simulink model "ParallelAndSeriesModulesSimulation"  (R2016a)
settings: Solver=VariableStepAuto  StartTime=0.0  StopTime=0.25  RelTol=1e-3
libraries: powerlib x17, powerlib_meascontrol x10, electricdrivelib x2
settings Model: Creator=kkfrk  LastModifiedBy=mesutto

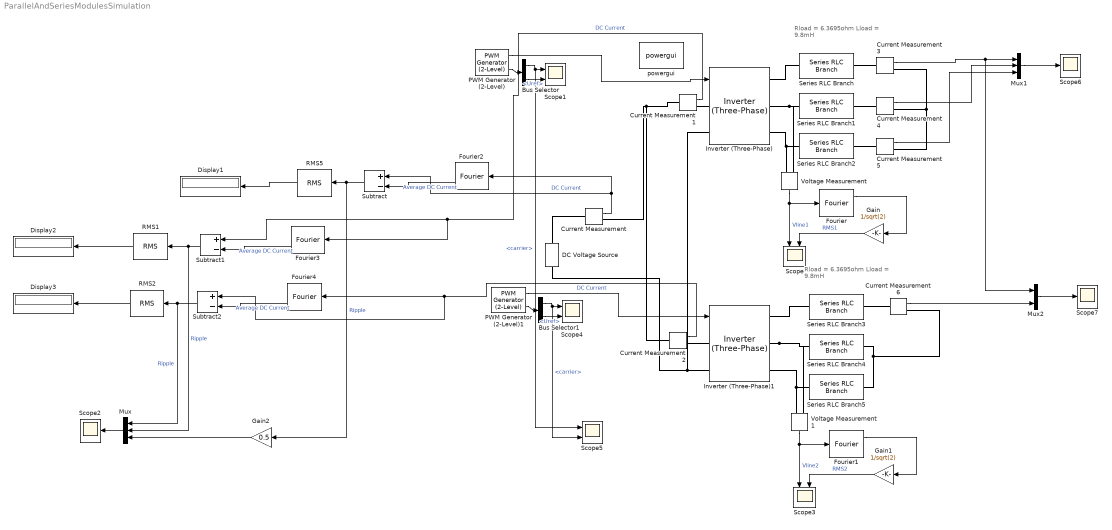
== system ParallelAndSeriesModulesSimulation ==
  note: Rload = 6.3695ohm
      | Lload = 9.8mH
  note: Rload = 6.3695ohm
      | Lload = 9.8mH
  Bus Selector : BusSelector  OutputSignals=carrier,Uref
  Bus Selector1 : BusSelector  OutputSignals=carrier,Uref
  Current Measurement{,1..6} (7 alike) : powerlib/Measurements/Current Measurement  PhasorSimulation=off  OutputType=Complex  PSBequivalent=0
  DC Voltage Source : powerlib/Electrical Sources/DC Voltage Source  Amplitude=400  Measurements=None
  Display1 : Display
  Display2 : Display
  Display3 : Display
  Fourier : powerlib_meascontrol/Measurements/Fourier  Freq=50  n=1  InInit=[0, 0]  Ts=0
  Fourier1 : powerlib_meascontrol/Measurements/Fourier  Freq=50  n=1  InInit=[0, 0]  Ts=0
  Fourier2 : powerlib_meascontrol/Measurements/Fourier  Freq=50  n=0  InInit=[0, 0]  Ts=0
  Fourier3 : powerlib_meascontrol/Measurements/Fourier  Freq=50  n=0  InInit=[0, 0]  Ts=0
  Fourier4 : powerlib_meascontrol/Measurements/Fourier  Freq=50  n=0  InInit=[0, 0]  Ts=0
  Gain : Gain  Gain=1/sqrt(2)
  Gain1 : Gain  Gain=1/sqrt(2)
  Gain2 : Gain  Gain=0.5
  Inverter (Three-Phase) : electricdrivelib/Fundamental Drive Blocks/Inverter (Three-Phase)  OverrideUsingVariant=Detailed  detailLevel=Detailed  driveType=Field-oriented control  Ts=2e-6  SnubberResistance=10e3  SnubberCapacitance=inf  Device=IGBT / Diodes  Ron=1e-3  ForwardVoltages=[1.2,1.2]  GTOparameters=[1e-6,2e-6]  IGBTparameters=[1e-6,2e-6]  Measurements=All voltages and currents  converterType=Inverter  SourceFrequency=60  ReferenceFrame=Rotor  dqInductances=[8.5e-3,8.5e-3]  Inductance=8.5e-3  Ls=0  Resistance=0.2  Flux=0.175  Stator_sm=[2.01e-3,4.289e-4,4.477e-3,1.354e-3]  Stator_im=[14.85e-3,0.3027e-3]  Rotor=[9.295e-3,0.3027e-3]  Lm=10.46e-3  p=4
      settings: AttributesFormatString=%<BlockChoice>
  Inverter (Three-Phase)1 : electricdrivelib/Fundamental Drive Blocks/Inverter (Three-Phase)  OverrideUsingVariant=Detailed  detailLevel=Detailed  driveType=Field-oriented control  Ts=2e-6  SnubberResistance=10e3  SnubberCapacitance=inf  Device=IGBT / Diodes  Ron=1e-3  ForwardVoltages=[1.2,1.2]  GTOparameters=[1e-6,2e-6]  IGBTparameters=[1e-6,2e-6]  Measurements=All voltages and currents  converterType=Inverter  SourceFrequency=60  ReferenceFrame=Rotor  dqInductances=[8.5e-3,8.5e-3]  Inductance=8.5e-3  Ls=0  Resistance=0.2  Flux=0.175  Stator_sm=[2.01e-3,4.289e-4,4.477e-3,1.354e-3]  Stator_im=[14.85e-3,0.3027e-3]  Rotor=[9.295e-3,0.3027e-3]  Lm=10.46e-3  p=4
      settings: AttributesFormatString=%<BlockChoice>
  Mux : Mux  Inputs=3
  Mux1 : Mux  Inputs=3
  Mux2 : Mux  Inputs=2
  PWM Generator (2-Level) : powerlib_meascontrol/Pulse & Signal Generators/PWM Generator (2-Level)  ModulatorType=Three-phase bridge (6 pulses)  ModulatorMode=Unsynchronized  Fc=1000  Pc=0  nF=27  MinMax="[ -1  1 ]"  SamplingTechnique=Natural  ModulatingSignals=on  m=0.8  Freq=50  Phase=0  Ts=0  ShowCarrierOutport=on
  PWM Generator (2-Level)1 : powerlib_meascontrol/Pulse & Signal Generators/PWM Generator (2-Level)  ModulatorType=Three-phase bridge (6 pulses)  ModulatorMode=Unsynchronized  Fc=1000  Pc=90  nF=27  MinMax="[ -1  1 ]"  SamplingTechnique=Natural  ModulatingSignals=on  m=0.8  Freq=50  Phase=0  Ts=0  ShowCarrierOutport=on
  RMS1 : powerlib_meascontrol/Measurements/RMS  TrueRMS=on  Freq=50  RMSInit=25  Ts=10e-6
  RMS2 : powerlib_meascontrol/Measurements/RMS  TrueRMS=on  Freq=50  RMSInit=25  Ts=10e-6
  RMS5 : powerlib_meascontrol/Measurements/RMS  TrueRMS=on  Freq=50  RMSInit=25  Ts=10e-6
  Scope{,1,3..5} (5 alike) : Scope  NumInputPorts=2
  Scope2 : Scope
  Scope6 : Scope
  Scope7 : Scope
  Series RLC Branch{,1..5} (6 alike) : powerlib/Elements/Series RLC Branch  LConnTagsString=__new0  RConnTagsString=__new0  BranchType=RLC  Resistance=6.3695  Inductance=9.8e-3  SetiL0=off  InitialCurrent=0  Capacitance=0  Setx0=off  InitialVoltage=0  Measurements=None
  Subtract : Sum  Inputs=+-
  Subtract1 : Sum  Inputs=+-
  Subtract2 : Sum  Inputs=+-
  Voltage Measurement : powerlib/Measurements/Voltage Measurement  PhasorSimulation=off  OutputType=Complex  PSBequivalent=0
  Voltage Measurement1 : powerlib/Measurements/Voltage Measurement  PhasorSimulation=off  OutputType=Complex  PSBequivalent=0
  powergui : powerlib/powergui  Priority=1  SimulationMode=Discrete  SolverType=Tustin/Backward Euler (TBE)  SampleTime=10e-6  frequency=60  SPID=off  DisableSnubberDevices=off  DisableRonSwitches=off  DisableVfSwitches=off  SwTol=0  DisplayEquations=off  Interpol=off  ExternalGateDelay=off  methode=off  Ts=10  FunctionMessages=off  echomessages=off  HookPort=off  EnableUseOfTLC=off  x0status=blocks  frequencyindice=0  Pbase=100e6  ErrMax=1e-4  Iterations=50  UnitsV=kV  UnitsW=MW  buscounter=0  RestoreLinks=warning  ResistiveCurrentMeasurement=off  Frange=[0:2:500]  Ylog=off  Xlog=on  ShowGrid=off  save=off  variable=ZData  structure=0  ZoomFFT=off  StartTime=0.0  cycles=1  DisplayStyle=1  fundamental=60  FreqAxis=off  MaxFrequency=1000  frequencyindicesteady=1  RmsSteady=1  display=off
  wires:
  Voltage Measurement/1 -> Scope/1, Fourier/1  "Vline1"
  PWM Generator (2-Level)/1 -> Inverter (Three-Phase)/1
  PWM Generator (2-Level)/2 -> Bus Selector/1
  Bus Selector/1 -> Scope5/1, Scope1/1  "<carrier>"
  Bus Selector/2 -> Scope1/2  "<Uref>"
  Fourier/1 -> Gain/1
  Gain/1 -> Scope/2  "RMS1"
  Voltage Measurement1/1 -> Fourier1/1, Scope3/1  "Vline2"
  Fourier1/1 -> Gain1/1
  Gain1/1 -> Scope3/2  "RMS2"
  Current Measurement/1 -> Subtract/1, Fourier2/1  "DC Current"
  PWM Generator (2-Level)1/1 -> Inverter (Three-Phase)1/1
  PWM Generator (2-Level)1/2 -> Bus Selector1/1
  Bus Selector1/1 -> Scope5/2, Scope4/1  "<carrier>"
  Bus Selector1/2 -> Scope4/2  "<Uref>"
  Fourier2/1 -> Subtract/2  "Average DC Current"
  Subtract/1 -> Gain2/1, RMS5/1  "Ripple"
  RMS5/1 -> Display1/1
  Current Measurement1/1 -> Fourier3/1, Subtract1/1  "DC Current"
  Fourier3/1 -> Subtract1/2  "Average DC Current"
  Subtract1/1 -> Mux/2, RMS1/1  "Ripple"
  RMS1/1 -> Display2/1
  Current Measurement2/1 -> Subtract2/1, Fourier4/1  "DC Current"
  Fourier4/1 -> Subtract2/2  "Average DC Current"
  Subtract2/1 -> Mux/1, RMS2/1  "Ripple"
  RMS2/1 -> Display3/1
  Mux/1 -> Scope2/1
  Mux1/1 -> Scope6/1
  Current Measurement3/1 -> Mux2/1, Mux1/1
  Current Measurement4/1 -> Mux1/2
  Current Measurement5/1 -> Mux1/3
  Mux2/1 -> Scope7/1
  Current Measurement6/1 -> Mux2/2
  Gain2/1 -> Mux/3
  connections:
  Series RLC Branch/LConn1 -- Inverter (Three-Phase)/RConn1
  Inverter (Three-Phase)/RConn3 -- Series RLC Branch2/LConn1 -- Voltage Measurement/LConn1
  Series RLC Branch1/LConn1 -- Inverter (Three-Phase)/RConn2 -- Voltage Measurement/LConn2
  Series RLC Branch5/LConn1 -- Voltage Measurement1/LConn1 -- Inverter (Three-Phase)1/RConn3
  Inverter (Three-Phase)1/RConn2 -- Series RLC Branch4/LConn1 -- Voltage Measurement1/LConn2
  Series RLC Branch4/RConn1 -- Current Measurement6/RConn1 -- Series RLC Branch5/RConn1
  Series RLC Branch3/LConn1 -- Inverter (Three-Phase)1/RConn1
  DC Voltage Source/RConn1 -- Current Measurement/LConn1
  Current Measurement/RConn1 -- Current Measurement2/LConn1 -- Current Measurement1/LConn1
  Inverter (Three-Phase)1/LConn2 -- Inverter (Three-Phase)/LConn2 -- DC Voltage Source/LConn1
  Current Measurement1/RConn1 -- Inverter (Three-Phase)/LConn1
  Current Measurement2/RConn1 -- Inverter (Three-Phase)1/LConn1
  Current Measurement3/LConn1 -- Series RLC Branch/RConn1
  Current Measurement4/LConn1 -- Series RLC Branch1/RConn1
  Current Measurement5/LConn1 -- Series RLC Branch2/RConn1
  Current Measurement3/RConn1 -- Current Measurement5/RConn1 -- Current Measurement4/RConn1
  Current Measurement6/LConn1 -- Series RLC Branch3/RConn1
